simulink model "acc_aeb"  (R2024b)
settings: Solver=FixedStepDiscrete  StartTime=0.0  StopTime=60  FixedStep=0.02  RelTol=1e-3
model workspace (MAT data in the model file):
  memory_initial = [0; 0; 5.5555555556; 0]
  scenario_input = [0 0.02 0.04 0.06 0.08 0.1 0.12 0.14 0.16 0.18 0.2 0.22 ... (12004 elements, 3001x4)]
  vehicle_initial = [22.2222222222; 22.2222222222; 45; 0]
(part 2 of 2)

== matlab function acc_aeb/Vehicle dynamics ==
  data: vehicle input; u input; next output; leadAcceleration input
function next = f(vehicle,u,leadAcceleration)
%#codegen
next = acc_plant(vehicle,u,leadAcceleration,0.02,0.25);
end

== matlab function acc_aeb/Supervisor and PID ==
  data: vehicle input; u output; memory input; present input; setSpeed input; next output; desired output; reference output; ttc output
function [u,next,desired,reference,ttc] = f(vehicle,memory,present,setSpeed)
%#codegen
p.dt = 0.02;
p.standstill_gap = 5;
p.headway = 1.5;
p.accel_max = 2;
p.brake_max = 4;
p.lead_brake_assumption = 6;
p.actuator_tau = 0.25;
p.jerk_limit = 2.5;
p.gap_gain = 0.20000000000000001;
p.kp = 0.80000000000000004;
p.ki = 0.12;
p.kd = 0.080000000000000002;
p.derivative_tau = 0.20000000000000001;
p.integral_limit = 10;
p.follow_enter_margin = 8;
p.follow_exit_margin = 18;
p.ttc_trigger = 1.5;
p.emergency_margin = 2;
[u,next,desired,reference,ttc] = acc_controller(vehicle(1),vehicle(2),vehicle(3),present,setSpeed,vehicle(4),memory,p);
end

== matlab function acc_aeb/Measurements ==
  data: vehicle input; memory input; u input; y output; desired input; reference input; ttc input; present input
function y = f(vehicle,memory,u,desired,reference,ttc,present)
%#codegen
y = [vehicle(1);vehicle(2);vehicle(3);desired;u;vehicle(4);memory(1);present;reference;ttc];
end

== matlab function acc_aeb/Dashboard signals ==
  data: y input; speed_kmh output; gap_m output; accel_mps2 output; mode output
function [speed_kmh,gap_m,accel_mps2,mode] = f(y)
%#codegen
speed_kmh = y(1:2)*3.6; gap_m = y(3:4); accel_mps2 = y(5:6); mode = y(7);
end
